simulink model "display_module_v1"  (R2025b)
settings: Solver=VariableStepAuto  StartTime=0.0  StopTime=10.0  RelTol=1e-3
libraries: aerolibanim x2, slctrl_linear x2, uavutilslib x1
settings Model: Creator=rosette-nebula  LastModifiedBy=rosette-nebula

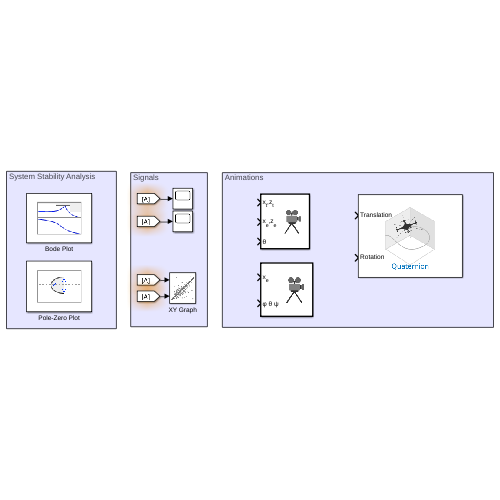
[thumbnail: Simulink's stored preview of the top-level diagram]
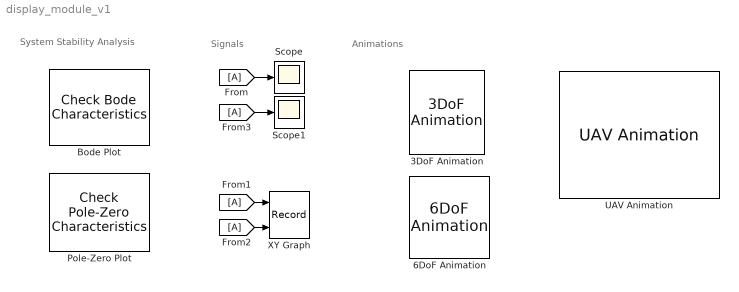
== system display_module_v1 ==
  note: Animations
  note: Signals
  note: System Stability Analysis
  3DoF Animation : aerolibanim/3DoF Animation  u1=[0 5000 -2000 2000 -5050 -3050]  u2=0.05  u3=1.0  u5=Fixed position  u6=[2000 500 -3150]  u7=10  u8=on
  6DoF Animation : aerolibanim/6DoF Animation  u1=[0 4000 -2000 2000 -5000 -3000]  u2=0.1  u3=1.0  u4=[4000 0 -5000]  u5=Fixed position  u6=[2000 500 -3150]  u7=10  u8=on
  Bode Plot : slctrl_linear/Check Bode  Characteristics  InstantiateOnLoad=on  SaveOperatingPoints=off  LinearizationIOs={}  LinearizeAt=SnapshotTimes  SnapshotTimes=[0]  TriggerType=rising  SampleTime=auto  RateConversionMethod=zoh  PreWarpFreq=10  UseExactDelayModel=off  UseFullBlockNameLabels=off  UseBusSignalLabels=off  enabled=on  stopWhenAssertionFail=off  export=off  ViewDlgPos=[]  OpenViewOnLoad=off  LaunchViewOnOpen=off  FrequencyUnits=rad/s  MagnitudeUnits=dB  PhaseUnits=deg  TimeUnits=seconds  EnableUpperBound=off  UpperBoundFrequencies=[]  UpperBoundMagnitudes=[]  EnableLowerBound=off  LowerBoundFrequencies=[]  LowerBoundMagnitudes=[]
      settings: LibrarySourceBlock=slctrlblks/Linear Analysis Plots/Bode Plot  SaveToWorkspace=off  SaveName=sys
  From{,1..3} (4 alike) : From
  Pole-Zero Plot : slctrl_linear/Check Pole-Zero Characteristics  InstantiateOnLoad=on  SaveOperatingPoints=off  LinearizationIOs={}  LinearizeAt=SnapshotTimes  SnapshotTimes=[0]  TriggerType=rising  SampleTime=auto  RateConversionMethod=zoh  PreWarpFreq=10  UseExactDelayModel=off  UseFullBlockNameLabels=off  UseBusSignalLabels=off  enabled=on  stopWhenAssertionFail=off  export=off  ViewDlgPos=[]  LaunchViewOnOpen=off  OpenViewOnLoad=off  FrequencyUnits=rad/s  MagnitudeUnits=dB  PhaseUnits=deg  TimeUnits=seconds  EnableSettlingTime=off  SettlingTime=[]  EnablePercentOvershoot=off  PercentOvershoot=[]  EnableDampingRatio=off  DampingRatio=[]  EnableNaturalFrequency=off  NaturalFrequencyBound=>=  NaturalFrequency=[]
      settings: LibrarySourceBlock=slctrlblks/Linear Analysis Plots/Pole-Zero Plot  SaveToWorkspace=off  SaveName=sys
  Scope : Scope
  Scope1 : Scope
  UAV Animation : uavutilslib/UAV Animation  NumUAV=1  DynamicUAVConfig=off  UAVType=Multirotor  UAVSize=1  UAVColor=[1 0 0]  UAVTrajectoryAlpha=1  InertialZDirection=Down  RotationFormat=Quaternion  DrawMarkers=off  SampleTime=-1
  XY Graph : Record  NumPorts=2.0  FileSettingsInternal="{\"entries\":[{\"content\":{\"excelSettings\":{\"content\":{},\"type\":\"Streamout.ExcelSettings\"},\"parquetSettings\":{\"content\":{},\"type\":\"Streamout.ParquetSettings\"}},\"type\":\"Streamout.FileSettingStorage\",\"uuid\":\"\"}],\"packageUris\":[\"http:\\/\\/schema.mathworks.com\\/mf0\\/streamout_blocks\\/R2020a\"],\"version\":\"1.0\"}"  FrameSettings=[0, 0]  Layout=[1 1]  SignalsInternal="{\"entries\":[{\"content\":{\"signals\":[{\"content\":{\"blockPath\":[],\"dimensions\":[1],\"domain\":\"\",\"lineColor\":\"#a2142f\",\"plots\":[ 1 ],\"port\":1,\"signalID\":1,\"signalName\":\"XY Graph:1\"},\"type\":\"RecordBlkView.Signal\",\"uuid\":\"\"},{\"content\":{\"blockPath\":[],\"dimensions\":[1],\"domain\":\"\",\"lineColor\":\"#139fff\",\"plots\":[ 1 ],\"port\":2,\"signalID\":2,\"signalName\":\"XY Graph:2\"},\"type\":\"RecordBlkView.Signal\",\"uuid\":\"\"}]},\"type\":\"RecordBlkView.InputSignals\",\"uuid\":\"\"}],\"packageUris\":[\"http:\\/\\/schema.mathworks.com\\/mf0\\/streamout_blocks\\/R2020a\"],\"version\":\"1.0\"}"  VisualizationBindings="{\"xyplotplugin\":{\"info\":[{\"series\":[{\"bindingParametersList\":[{\"parameter\":\"X-Axis\",\"signalID\":1,\"signalName\":\"XY Graph:1\"},{\"parameter\":\"Y-Axis\",\"signalID\":2,\"signalName\":\"XY Graph:2\"}],\"seriesID\":0}],\"subplotID\":1}]}}"  CompatibilityTag=XY
  wires:
  From/1 -> Scope/1
  From1/1 -> XY Graph/1
  From2/1 -> XY Graph/2
  From3/1 -> Scope1/1
